simulink library "uavsimBlockset_DerivedAerodynamicConditions"  (Simulink 8.0)
settings: Solver=ode45  StartTime=0.0  StopTime=10.0  RelTol=1e-3
libraries: aerolibasang x3
settings Model: Creator=mstolle  LastModifiedBy=j.bolting

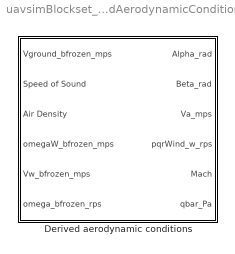
== system uavsimBlockset_DerivedAerodynamicConditions ==
  Derived aerodynamic conditions : Subsystem

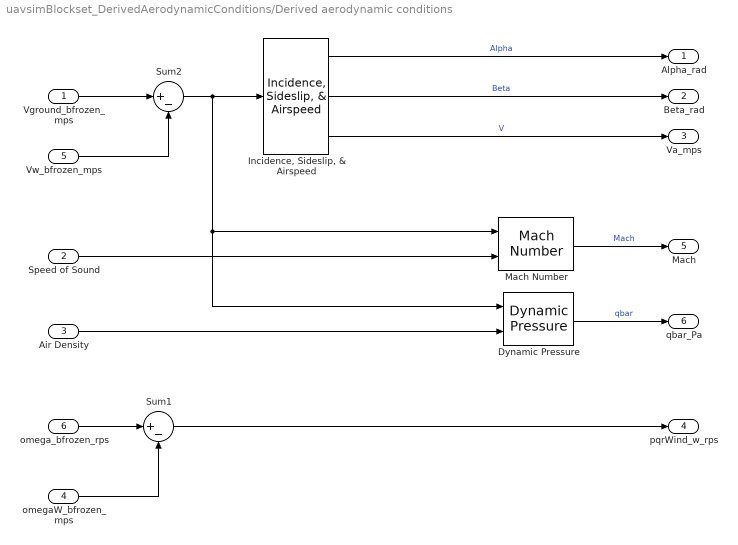
== system uavsimBlockset_DerivedAerodynamicConditions/Derived aerodynamic conditions ==
  Vground_bfrozen_mps : Inport  PortDimensions=3
  Speed of Sound : Inport  Port=2
  Air Density : Inport  Port=3
  omegaW_bfrozen_mps : Inport  Port=4  PortDimensions=3
  Vw_bfrozen_mps : Inport  Port=5  PortDimensions=3
  omega_bfrozen_rps : Inport  Port=6  PortDimensions=3
  Dynamic Pressure : aerolibasang/Dynamic Pressure
  "Incidence, Sideslip, & Airspeed" : aerolibasang/Incidence, Sideslip, & Airspeed
  Mach Number : aerolibasang/Mach Number
  Sum1 : Sum  Inputs=|+-  SaturateOnIntegerOverflow=on  InputSameDT=on  OutDataTypeStr=Inherit: Same as first input
  Sum2 : Sum  Inputs=|+-  SaturateOnIntegerOverflow=on  InputSameDT=on  OutDataTypeStr=Inherit: Same as first input
  Alpha_rad : Outport
  Beta_rad : Outport  Port=2
  Va_mps : Outport  Port=3
  "pqrWind_w_rps " : Outport  Port=4
  Mach : Outport  Port=5
  qbar_Pa : Outport  Port=6  InitialOutput=0
  wires:
  Vw_bfrozen_mps/1 -> Sum2/2
  Sum2/1 -> "Incidence, Sideslip, & Airspeed"/1, Mach Number/1, Dynamic Pressure/1
  Vground_bfrozen_mps/1 -> Sum2/1
  Speed of Sound/1 -> Mach Number/2
  "Incidence, Sideslip, & Airspeed"/3 -> Va_mps/1  "V"
  Dynamic Pressure/1 -> qbar_Pa/1  "qbar"
  Mach Number/1 -> Mach/1  "Mach"
  "Incidence, Sideslip, & Airspeed"/1 -> Alpha_rad/1  "Alpha"
  "Incidence, Sideslip, & Airspeed"/2 -> Beta_rad/1  "Beta"
  Air Density/1 -> Dynamic Pressure/2
  omega_bfrozen_rps/1 -> Sum1/1
  omegaW_bfrozen_mps/1 -> Sum1/2
  Sum1/1 -> "pqrWind_w_rps "/1
